simulink model "Sterowanie_StatkiemORDI_2015"  (R2015b)
settings: Solver=FixedStepAuto  SolverMode=SingleTasking  StartTime=0.0  StopTime=10  FixedStep=0.001  MaxStep=0.01  MinStep=.009  RelTol=1e-2
settings Model: Creator=szymo  LastModifiedBy=szymo
settings SolverCC: AlgebraicLoopSolver=LineSearch
settings DataIOCC: LimitDataPoints=off  ReturnWorkspaceOutputs=on
settings DebuggingCC: AllowSymbolicDim=on  SFUnexpectedBacktrackingDiag=error  SFNoUnconditionalDefaultTransitionDiag=error
settings ModelReferenceCC: PropagateSignalLabelsOutOfModel=on
settings SFSimCC: SimUseLocalCustomCode=on
settings RTWCC: RTWUseLocalCustomCode=on
settings GRTTargetCC: TargetLangStandard=C99 (ISO)
settings ConfigComp: CovMetricSettings=dwe  CovHtmlReporting=off  CovSaveCumulativeToWorkspaceVar=off  CovSaveSingleToWorkspaceVar=off  CovModelRefEnable=Off  CovExternalEMLEnable=on

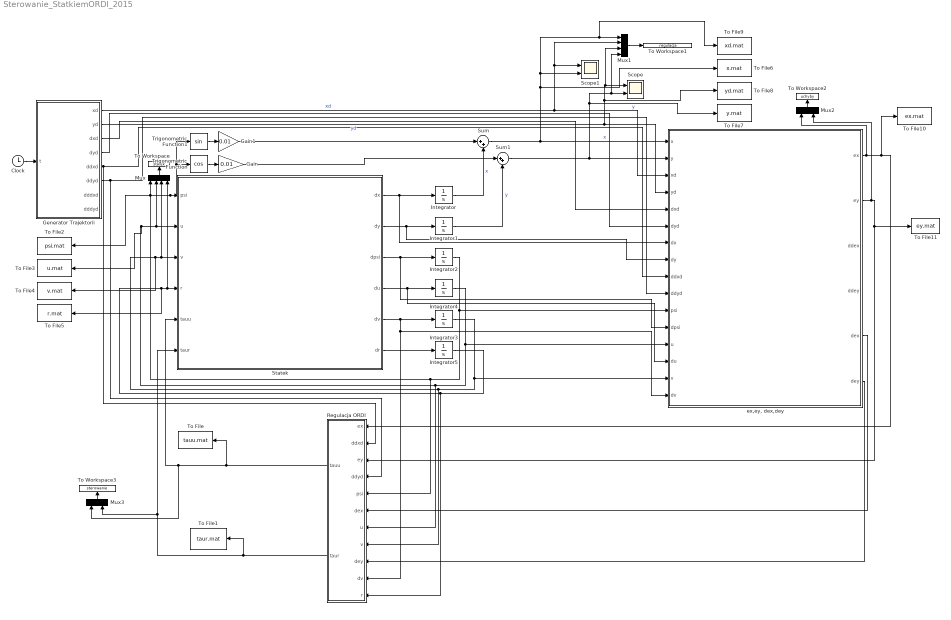
== system Sterowanie_StatkiemORDI_2015 ==
  Clock : Clock
  Gain : Gain  Gain=0.01
  Gain1 : Gain  Gain=0.01
  Generator Trajektorii : MATLAB Function  TreatAsAtomicUnit=on
  Integrator : Integrator  InitialCondition=-0.01
  Integrator1 : Integrator  InitialCondition=1.01
  Integrator2 : Integrator  InitialCondition=0.01
  Integrator3 : Integrator  InitialCondition=0.1
  Integrator4 : Integrator  InitialCondition=0.1
  Integrator5 : Integrator  InitialCondition=0.1
  Mux : Mux
  Mux1 : Mux
  Mux2 : Mux  Inputs=2
  Mux3 : Mux  Inputs=2
  Regulacja ORDI : Subsystem
  Scope : Scope  NumInputPorts=2
  Scope1 : Scope  NumInputPorts=2
  Statek : MATLAB Function  TreatAsAtomicUnit=on
  Sum : Sum  Inputs=|++
  Sum1 : Sum  Inputs=|++
  To File : ToFile  Filename=tauu.mat  SaveFormat=Timeseries
  To File1 : ToFile  Filename=taur.mat  SaveFormat=Timeseries
  To File10 : ToFile  Filename=ex.mat  SaveFormat=Timeseries
  To File11 : ToFile  Filename=ey.mat  SaveFormat=Timeseries
  To File2 : ToFile  Filename=psi.mat  SaveFormat=Timeseries
  To File3 : ToFile  Filename=u.mat  SaveFormat=Timeseries
  To File4 : ToFile  Filename=v.mat  SaveFormat=Timeseries
  To File5 : ToFile  Filename=r.mat  SaveFormat=Timeseries
  To File6 : ToFile  Filename=x.mat  SaveFormat=Timeseries
  To File7 : ToFile  Filename=y.mat  SaveFormat=Timeseries
  To File8 : ToFile  Filename=yd.mat  SaveFormat=Timeseries
  To File9 : ToFile  Filename=xd.mat  SaveFormat=Timeseries
  To Workspace : ToWorkspace  VariableName=statek  SaveFormat=Timeseries  SampleTime=-1
  To Workspace1 : ToWorkspace  VariableName=regulacja  SaveFormat=Timeseries  SampleTime=-1
  To Workspace2 : ToWorkspace  VariableName=uchyby  SaveFormat=Timeseries  SampleTime=-1
  To Workspace3 : ToWorkspace  VariableName=sterowanie  SaveFormat=Timeseries  SampleTime=-1
  Trigonometric Function : Trigonometry  Operator=cos
  Trigonometric Function1 : Trigonometry
  "ex,ey, dex,dey" : MATLAB Function  TreatAsAtomicUnit=on
  wires:
  Clock/1 -> Generator Trajektorii/1(t)
  Trigonometric Function/1 -> Gain/1
  Trigonometric Function1/1 -> Gain1/1
  Statek/2(dy) -> "ex,ey, dex,dey"/8(dy), Integrator1/1
  Statek/3(dpsi) -> "ex,ey, dex,dey"/12(dpsi), Integrator2/1
  Statek/4(du) -> "ex,ey, dex,dey"/14(du), Integrator4/1
  Statek/6(dr) -> Integrator5/1
  Gain1/1 -> Sum/1
  Gain/1 -> Sum1/1
  Integrator/1 -> Sum/2  "x"
  Integrator1/1 -> Sum1/2  "y"
  Sum/1 -> "ex,ey, dex,dey"/1(x), To File6/1, To File9/1, Mux1/1, Scope1/2  "x"
  Sum1/1 -> To File7/1, Mux1/4, Scope/2, "ex,ey, dex,dey"/2(y)  "y"
  Generator Trajektorii/2(yd) -> To File8/1, Mux1/3, Scope/1, "ex,ey, dex,dey"/4(yd)  "yd"
  Generator Trajektorii/5(ddxd) -> Regulacja ORDI/2(ddxd), "ex,ey, dex,dey"/9(ddxd)
  Generator Trajektorii/6(ddyd) -> Regulacja ORDI/4(ddyd), "ex,ey, dex,dey"/10(ddyd)
  Generator Trajektorii/3(dxd) -> "ex,ey, dex,dey"/5(dxd)
  Generator Trajektorii/4(dyd) -> "ex,ey, dex,dey"/6(dyd)
  Statek/1(dx) -> "ex,ey, dex,dey"/7(dx), Integrator/1
  "ex,ey, dex,dey"/1(ex) -> To File10/1, Regulacja ORDI/1(ex), Mux2/1
  "ex,ey, dex,dey"/2(ey) -> Mux2/2, To File11/1, Regulacja ORDI/3(ey)
  Integrator2/1 -> "ex,ey, dex,dey"/11(psi), Trigonometric Function/1, Trigonometric Function1/1, Statek/1(psi), To File2/1, Mux/1, Regulacja ORDI/5(psi)
  "ex,ey, dex,dey"/5(dex) -> Regulacja ORDI/6(dex)
  "ex,ey, dex,dey"/6(dey) -> Regulacja ORDI/9(dey)
  Integrator4/1 -> "ex,ey, dex,dey"/13(u), Regulacja ORDI/7(u), To File3/1, Mux/2, Statek/2(u)
  Integrator3/1 -> "ex,ey, dex,dey"/15(v), Regulacja ORDI/8(v), To File4/1, Mux/3, Statek/3(v)
  Statek/5(dv) -> Regulacja ORDI/10(dv), "ex,ey, dex,dey"/16(dv), Integrator3/1
  Integrator5/1 -> Regulacja ORDI/11(r), To File5/1, Statek/4(r), Mux/4
  Generator Trajektorii/1(xd) -> "ex,ey, dex,dey"/3(xd), Mux1/2, Scope1/1  "xd"
  Mux/1 -> To Workspace/1
  Mux1/1 -> To Workspace1/1
  Mux2/1 -> To Workspace2/1
  Mux3/1 -> To Workspace3/1
  Regulacja ORDI/1(tauu) -> Mux3/1, Statek/5(tauu), To File/1
  Regulacja ORDI/2(taur) -> To File1/1, Mux3/2, Statek/6(taur)

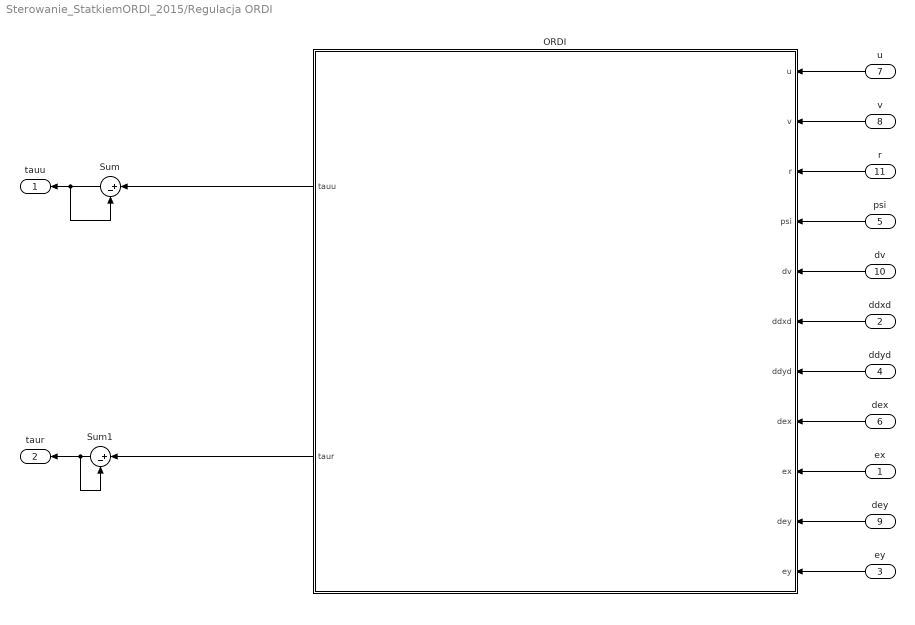
== system Sterowanie_StatkiemORDI_2015/Regulacja ORDI ==
  ex : Inport
  ddxd : Inport  Port=2
  ey : Inport  Port=3
  ddyd : Inport  Port=4
  psi : Inport  Port=5
  dex : Inport  Port=6
  u : Inport  Port=7
  v : Inport  Port=8
  dey : Inport  Port=9
  dv : Inport  Port=10
  r : Inport  Port=11
  ORDI : MATLAB Function  TreatAsAtomicUnit=on
  Sum : Sum  Inputs=|+-
  Sum1 : Sum  Inputs=|+-
  tauu : Outport
  taur : Outport  Port=2
  wires:
  dey/1 -> ORDI/10(dey)
  dv/1 -> ORDI/5(dv)
  ey/1 -> ORDI/11(ey)
  r/1 -> ORDI/3(r)
  v/1 -> ORDI/2(v)
  ex/1 -> ORDI/9(ex)
  u/1 -> ORDI/1(u)
  psi/1 -> ORDI/4(psi)
  ddyd/1 -> ORDI/7(ddyd)
  ddxd/1 -> ORDI/6(ddxd)
  dex/1 -> ORDI/8(dex)
  ORDI/1(tauu) -> Sum/1
  Sum/1 -> Sum/2, tauu/1
  ORDI/2(taur) -> Sum1/1
  Sum1/1 -> taur/1, Sum1/2

== matlab function Sterowanie_StatkiemORDI_2015/Generator Trajektorii ==
  data: t input; xd output; yd output; dxd output; dyd output; ddxd output; ddyd output; dddxd output; dddyd output
function [xd,yd,dxd,dyd,ddxd,ddyd,dddxd,dddyd] = fcn(t)

xd = sin(t);
yd = cos(t);
dxd=cos(t);
dyd=-sin(t);
ddxd = -sin(t);
ddyd = -cos(t);
dddxd = -cos(t);
dddyd = sin(t);

== matlab function Sterowanie_StatkiemORDI_2015/Statek ==
  data: psi input size=1; u input size=1; v input size=1; dx output size=1; r input size=1; dy output size=1; dpsi output size=1; du output size=1; dv output size=1; dr output size=1; tauu input size=1; taur input size=1
function [dx,dy,dpsi,du,dv,dr] = fcn(psi,u,v,r,tauu,taur)
m11=1.956;
m22=2.405;
m33=0.043;
d11=2.436;
d22=12.992;
d33=0.0564;
dx = u*cos(psi)-v*sin(psi);
dy = u*sin(psi)+v*cos(psi);
dpsi = r;
du = (m22*v*r-d11*u+tauu)/m11;
dv = (-m11*u*r-d22*v)/m22;
dr = ((m11-m22)*u*v-d33*r+taur)/m33;

== matlab function Sterowanie_StatkiemORDI_2015/ex,ey, dex,dey ==
  data: x input; y input; xd input; yd input; dxd input; dyd input; dx input; dy input; ddxd input; ddyd input; psi input; dpsi input; u input; du input; v input; dv input; ex output; ey output; ddex output; ddey output; dex output; dey output
function [ex,ey,ddex,ddey,dex,dey] = fcn(x,y,xd,yd,dxd,dyd,dx,dy,ddxd,ddyd,psi,dpsi,u,du,v,dv)

ex = x-xd;
ey = y-yd;
m11=1.956;
dex=dx-dxd;
dey=dy-dyd;
ddex = du*cos(psi)-u*dpsi*sin(psi)-dv*sin(psi)-v*dpsi*cos(psi)-ddxd;
ddey = du*sin(psi)+u*dpsi*cos(psi)+dv*cos(psi)-v*dpsi*sin(psi)-ddyd;

== matlab function Sterowanie_StatkiemORDI_2015/Regulacja ORDI/ORDI ==
  data: u input; tauu output; v input; r input; psi input; dv input; ddxd input; ddyd input; dex input; ex input; dey input; ey input; taur output
function [tauu,taur] = fcn(u,v,r,psi,dv,ddxd,ddyd,dex,ex,dey,ey)
m11=1.956;
m22=2.405;
m33=0.043;
d11=2.436;
d22=12.992;
d33=0.0564;
k31=4;
k32=4;
k33=4;
k34=4;
l=0.01;

fu = (m22*v*r-d11*u)/m11;
fr = ((m11-m22)*u*v-d33*r)/m33;
F = [fu*cos(psi)-u*r*sin(psi)-dv*sin(psi)-v*r*cos(psi)-ddxd;fu*sin(psi)+u*r*cos(psi)+dv*cos(psi)-v*r*sin(psi)-ddyd];
F3 = F + [-l*fr*sin(psi) - l*r^2*cos(psi);l*fr*cos(psi)-l*r^2*sin(psi)];
G3 = [cos(psi)/m11, -l*sin(psi)/m33; sin(psi)/m11, l*cos(psi)/m33];
wek = (G3)^(-1)*(-1*F3+[-k31*dex-k32*ex; -k33*dey - k34*ey]);
tauu = wek(1);
taur = wek(2);
